simulink model "Discrete_system_state_space_realization"  (Simulink 7.6)
settings: Solver=ode45  StartTime=0.0  StopTime=10.0  RelTol=1e-3
settings Model: Creator=administrator  LastModifiedBy=administrator

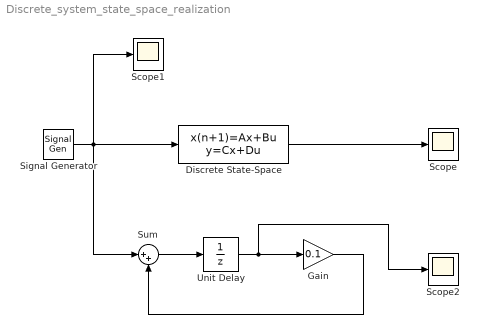
== system Discrete_system_state_space_realization ==
  Discrete State-Space : DiscreteStateSpace  A=0.1  D=0
  Gain : Gain  Gain=0.1
  Scope : Scope
  Scope1 : Scope
  Scope2 : Scope
      settings: SaveName=ScopeData2
  Signal Generator : SignalGenerator  WaveForm=square  Frequency=0.5
  Sum : Sum  Inputs=|++
  Unit Delay : UnitDelay
  wires:
  Signal Generator/1 -> Discrete State-Space/1, Scope1/1, Sum/1
  Discrete State-Space/1 -> Scope/1
  Unit Delay/1 -> Gain/1, Scope2/1
  Gain/1 -> Sum/2
  Sum/1 -> Unit Delay/1
